simulink model "rtvdp"  (Simulink 6.0)
settings: Solver=ode4  StartTime=0.0  StopTime=10.0  RelTol=1e-3
settings Model: Creator=Houska  LastModifiedBy=Houska  ExtModeMexFile=rtwinext  ProdHWDeviceType=32-bit Real-Time Windows Target
settings ConfigSet: SimulationMode=external
settings DataIOCC: SaveOutput=off  SaveTime=off  SignalLoggingName=logsOut
settings OptimizationCC: MultiInstanced=off
settings FormatCC: IgnoreBidirectionalLines=off
settings HardwareCC: ProdIntDivRoundTo=Zero  ProdEndianess=LittleEndian  ProdHWDeviceType=32-bit Real-Time Windows Target
settings RTWCC: SystemTargetFile=rtwin.tlc  TemplateMakefile=rtwin.tmf  Description=Real-Time Windows Target  ProcessScript=rtwin_make_rtw_hook
settings CodeAppCC: SimulinkBlockComments=off
settings RTWinTargetCC: TargetFcnLib=iso_c_tmw.mat  CCOptimize=on

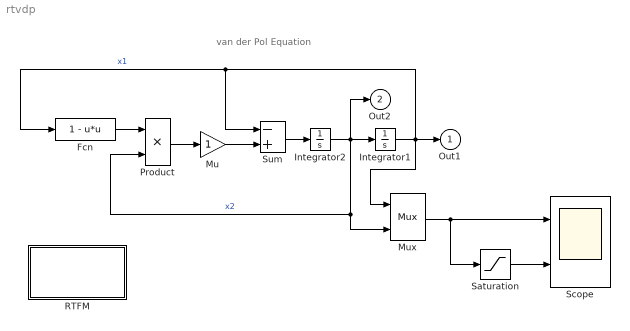
== system rtvdp ==
  note: van der Pol Equation
  Fcn : Fcn  Expr=1 - u*u
  Integrator1 : Integrator  InitialCondition=2
  Integrator2 : Integrator
  Mu : Gain  SaturateOnIntegerOverflow=on
  Mux : Mux  Inputs=2
  Product : Product  SaturateOnIntegerOverflow=on  InputSameDT=on
  "RTFM " : Subsystem
      mask Type: Frame-Based Simulation Info
      mask Display: disp('Info')
  Saturation : Saturate  UpperLimit=2  LowerLimit=-2
  Scope : Scope  NumInputPorts=2
      settings: TimeRange=10  YMin=-3~-5  YMax=5~5  DataFormat=Structure
  Sum : Sum  Inputs=-+  SaturateOnIntegerOverflow=on  InputSameDT=on
  Out1 : Outport  InitialOutput=0
  Out2 : Outport  Port=2  InitialOutput=0
  wires:
  Sum/1 -> Integrator2/1
  Integrator2/1 -> Out2/1, Integrator1/1, Product/2, Mux/2  "x2"
  Integrator1/1 -> Out1/1, Fcn/1, Sum/1, Mux/1  "x1"
  Product/1 -> Mu/1
  Mu/1 -> Sum/2
  Fcn/1 -> Product/1
  Saturation/1 -> Scope/2
  Mux/1 -> Saturation/1, Scope/1

== system rtvdp/RTFM  ==
  note: How to run this demo:
      |
      | 1) Build the model using Tools->Real-Time Workshop->Build Model.
      | 2) Connect to the real-time code using Simulation->Connect to target.
      | 3) Start the real-time execution using Simulation->Start real-time code.
